simulink model "Experiment_3_cs"  (Simulink 8.4)
settings: Solver=ode5  SolverMode=SingleTasking  StartTime=0.0  StopTime=inf  FixedStep=1/100  RelTol=1e-3
PreLoadFcn:
  | mbxruntime.callbacks.PreLoadFcn(bdroot);
PostLoadFcn:
  | mbxruntime.callbacks.PostLoadFcn(bdroot);
InitFcn:
  | mbxruntime.callbacks.InitFcn(bdroot);
StartFcn:
  | mbxruntime.callbacks.StartFcn(bdroot);
StopFcn:
  | mbxruntime.callbacks.StopFcn(bdroot);
undefined symbols (not defined in the file or in its folder): dfreq, gray, Rec, SDTV, strel
libraries: simulink x88, PreScanSimulinkLibrary x24, simulink_extras x22, visiontextngfix x15, visionconversions x3, PreScanUsefulBlocks x3, visionsinks x2, simulink_need_slupdate x2, visionstatistics x1, visionmorphops x1, visionanalysis x1
(part 2 of 12)

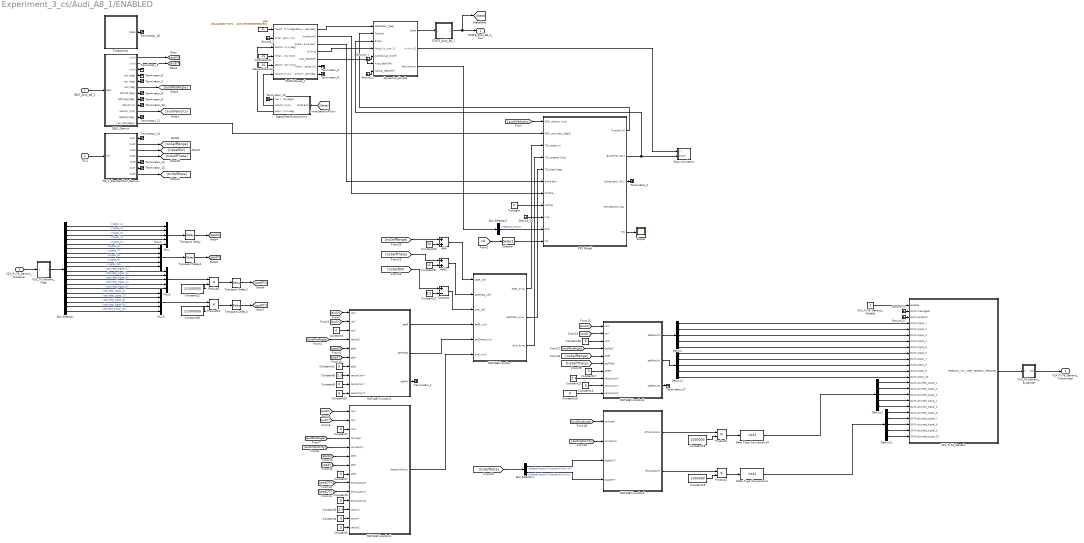
== system Experiment_3_cs/Audi_A8_1/ENABLED ==
  SELF_Audi_A8_1 : Inport  Tag=inport/SelfPort  OutDataTypeStr=Bus: PRESCAN_SELFSENSORDATA  PortDimensions=1  SampleTime=1/100  BusOutputAsStruct=on
  TIS_1 : Inport  Tag=inport/TIS  Port=2  OutDataTypeStr=Bus: PRESCAN_SCANNERSENSOR_MESSAGE  PortDimensions=5  SampleTime=1/50  BusOutputAsStruct=on
  V2X_Rx76_Generic_Receiver : Inport  Tag=inport/plugin/sfun_V2X_Generic_Receiver  Port=3  BusOutputAsStruct=on
  Add : Sum
  Add1 : Sum
  Bus Selector : BusSelector  OutputSignals=DATA.signal_1,DATA.signal_2,DATA.signal_3,DATA.signal_4,DATA.signal_5,DATA.signal_6,DATA.signal_7,DATA.signal_8,DATA.signal_9,DATA.signal_10,DATA.discrete_signal_1,DATA.discrete_signal_2,DATA.discrete_signal_3,DATA.discrete_signal_4,DATA.discrete_signal_5,DATA.discrete_signal_6,DATA.discrete_signal_7,DATA.discrete_signal_8,DATA.discrete_signal_9,DATA.discrete_signal_10
  Bus Selector1 : BusSelector  OutputSignals=DopplerVelocityTranslationX[ms-1],DopplerVelocityTranslationY[ms-1]
  Bus Selector2 : BusSelector  OutputSignals=NEngine_[rpm]
  Constant{,1..2,4..7,9..11,14..17} (14 alike) : Constant  Value=0
  Constant12 : Constant  Value=1/1000000
  Constant13 : Constant  Value=2.3
  Constant18 : Constant  Value=1000000
  Constant19 : Constant  Value=1000000
  Constant20 : Constant  Value=10
  Constant21 : Constant  Value=15
  Constant22 : Constant  Value=0.5
  Constant28 : Constant  Value=1/1000000
  Constant3 : Constant  Value=2.3
  Constant8 : Constant  Value=2.3
  Data Type Conversion1 : DataTypeConversion  OutDataTypeStr=int32
  Data Type Conversion10 : DataTypeConversion  OutDataTypeStr=int32
  Demux{,1..3} (4 alike) : Demux  Outputs=5
  DesiredVelocity : Constant  Tag=DesiredVelocity  Value=15
  Dynamics_Simple : Subsystem  Tag=Simple_Vehicle_Dynamics  mask(PreScan Block: Simple Dynamics){Migrate=on, TimeStep=1/100, ComputationMode=Continuous_Time}
      mask prompts: Migrate "Migrate. During migration this block will be replaced by a newer one."; TimeStep "Auto assigned: Time Step [s]"; ComputationMode "Computation mode:"
      mask help:
      | The Simple Dynamics Model is selected in the GUI to simulate vehicle dynamics behavior.
      |
      | The Simple Dynamics Model is completely open to the user. The parameters of this model can be set in the Simple Dynamics dialog in the GUI.
      |
      | For more information, please click Help.
      mask init:
      | p = SimpleDyn_pars;
      settings: DeleteFcn=PreScanBlockDeleteFcn;
      mask Help: eval('openHelp(220)')
      mask Display:
      | image(imread('SimpleDyn.png'))
      | port_label('input', 1, '{\delta}_S_t_ _e_e_r [deg]','texmode','on')
      | port_label('input', 2, 'Throttle [%]')
      | port_label('input', 3, 'Brake Pres [bar]')
      | port_label('input', 4, 'V_0 [ms-1]','texmode','on')
      | port_label('input', 5, 'Auto=[0]/Manual=[1]')
      | port_label('input', 6, 'Auto_GearShift')
      | port_label('input', 7, 'Manual_GearShift')
      | port_label('output', 1, 'State')
      | port_label('output', 2, 'Vx [ms-1]')
      | port_label('output', 3, 'Perf Params')
  Ground_{1..5,26} (6 alike) : Ground
  InitialVelocity : Constant  Tag=InitialVelocity  Value=15
  MATLAB Function : MATLAB Function  TreatAsAtomicUnit=on
  MATLAB Function1 : MATLAB Function  TreatAsAtomicUnit=on
  MATLAB Function2 : MATLAB Function  TreatAsAtomicUnit=on
  MATLAB Function3 : MATLAB Function  TreatAsAtomicUnit=on
  MATLAB Function4 : MATLAB Function  TreatAsAtomicUnit=on
  Mux{,1..3} (4 alike) : Mux  Inputs=5
  PPS Model : Subsystem  mask(PPS Model){MaxSpeed=70, MaxBrakePressure=150, BrakeDelay=100, LaneWidth=3.5, TISMaxRange=40, TISMaxTheta=60, TISfreq=25, TISdet=32, Camfreq=50, Mainfreq=100, DisplaySwitch=on, DisplayFreq=25, RadarSwitch=on, RadarFreq=25}
      mask prompts: MaxSpeed "Vehicle cut-off speed [km/h]"; MaxBrakePressure "Maximum value of braking pressure available [bar]"; BrakeDelay "Braking system delay [ms]"; LaneWidth "Lane width [m]"; TISMaxRange "TIS maximum range [m]"; TISMaxTheta "TIS maximum theta [deg]"; TISfreq "TIS frequency [Hz]"; TISdet "Max. number of Radar detected objects [-]"; Camfreq "Camera frequency [Hz]"; Mainfreq "Compilation sheet frequency [Hz]"; DisplaySwitch "Show EGO parameters visualization"; DisplayFreq "EGO parameters visualization frequency [Hz]"; RadarSwitch "Show radar visualization"; RadarFreq "Radar frequency [Hz]"
      mask help: PreScan Experiment and Pedestrian Protection System parameters
      mask Help: eval('openHelp(8130)')
      mask Callback DisplaySwitch:
      | en = get_param(gcb,'MaskEnables');
      | switch get_param(gcb, 'DisplaySwitch')
      |     case 'off'
      |         en{12} = 'off';
      |     case 'on'
      |         en{12} = 'on';
      | end
      | set_param(gcb,'MaskEnables',en);
      mask Callback RadarSwitch:
      | en = get_param(gcb,'MaskEnables');
      | switch get_param(gcb, 'RadarSwitch')
      |     case 'off'
      |         en{14} = 'off';
      |     case 'on'
      |         en{14} = 'on';
      | end
      | set_param(gcb,'MaskEnables',en);
  PathFollower_1 : Subsystem  Tag=pathFollower  mask(PreScan Block: Path Follower){Migrate=on, FileName='Trajectory_2.mat', TunableSteeringGain=1, XShifting_wrt_COG=0}
      mask prompts: Migrate "Migrate. During migration this block will be replaced by a newer one."; FileName "Trajectory Name"; TunableSteeringGain "TunableSteeringGain [-]"; XShifting_wrt_COG "XShifting_wrt_COG [m]"
      mask help:
      | The Path Follower Model is selected in the GUI to simulate driver behavior.
      |
      | For more information, please click Help.
      mask init:
      | load(['trajectories/',eval(FileName)])
      | traject=trajectory';
      | 
      | Traj_x=traject(:,2);
      | Traj_y=traject(:,3);
      | Traj_z=traject(:,4);
      | Traj_vx=traject(:,8);
      | Traj_vy=traject(:,9);
      | Traj_vz=traject(:,10);
      mask Help: eval('openHelp(232)')
  Product{1..3,12} (4 alike) : Product
  SELF_Demux : Subsystem  Tag=demux/SelfPort  mask(PreScan Demux Block:){}
      mask help:
      | The SELF port shows (state) information of the actor itself. The outputs are position in the experiment's axis system and the GPS coordinates, and the object's absolute velocity and compass heading.
      |
      | For more information, please click Help.
      settings: DeleteFcn=PreScanBlockDeleteFcn;
      mask Help: eval('openHelp(462)')
      mask Display:
      | port_label('output',1,'x [m]')
      | port_label('output',2,'y [m]')
      | port_label('output',3,'z [m]','texmode','on')
      | port_label('output',4,'Rotx [deg]','texmode','on')
      | port_label('output',5,'Roty [deg]','texmode','on')
      | port_label('output',6,'Rotz [deg]','texmode','on')
      | port_label('output',7,'GPS lat [deg]','texmode','on')
      | port_label('output',8,'GPS long [deg]','texmode','on')
      | port_label('output',9,'GPS alt [m]','texmode','on')
      | port_label('output',10,'Velocity [m/s]')
      | port_label('output',11,'Heading [deg]')
      | port_label('output',12,'Yaw rate [deg/s]')
  STATE_Audi_A8_1 : Subsystem  Tag=mux/StatePort  Priority=0  LoadFcn=load PrescanStateActuatorData  mask(PreScan Sink Block: State){x0=58.689357757568359, y0=151.23704528808594, z0=0.55, Roll0=0, Pitch0=0, Yaw0=359.99999999999295, TimeStep=1/100}
      mask prompts: x0 "Ini x-position VEHICLE wrt GLOBAL axis system [m]"; y0 "Ini y-position VEHICLE wrt GLOBAL axis system [m]"; z0 "Ini z-position VEHICLE wrt GLOBAL axis system [m]"; Roll0 "Ini roll-angle BODY wrt VEHICLE axis system [deg]"; Pitch0 "Ini pitch-angle BODY wrt VEHICLE axis system [deg]"; Yaw0 "Ini yaw-angle VEHICLE wrt GLOBAL axis system [deg]"; TimeStep "Auto-Assigned: Upload Period [s]"
      mask help:
      | The Actor State contains a vector signal of size (9x1), containing the following signals:
      |
      | -  Position                  (x,y,z)                                     [m]
      | -  Velocity                  (vx,vy,vz)                               [m/s]
      | -  Angles                    (Roll, Pitch, Yaw)                   [rad]
      |
      | The Actor state is defined in the global axis system.
      | The state is superponed on the Initial position defined in the GUI.
      |
      | For more information, please click Help.
      settings: DeleteFcn=PreScanBlockDeleteFcn;
      mask Help: eval('openHelp(222)')
      mask Display: image(imread('State.png'))
  Scope : Scope
  Selector : Selector  InputPortWidth=5
  State2PathFollowerCnv : Subsystem  Tag=State2PFConnection/cnv
  Stop simulation : Subsystem
  Subtract : Sum  Inputs=+-
  TIS_1_StandardCoh_Demux : Subsystem  Tag=demux/TIS/StandardCoh  TreatAsAtomicUnit=on  mask(PreScan Demux Block: TIS){MAXMESSAGES=5}
      mask prompts: MAXMESSAGES "Number of Objects"
      mask Help: eval('openHelp(449)')
      mask Display:
      | port_label('input',1,'TIS')
      | port_label('output',1,'Beam ID [-]')
      | port_label('output',2,'Range [m]')
      | port_label('output',3,'DopplerVelocity [m/s]')
      | port_label('output',4,'{\theta} [deg]','texmode','on')
      | port_label('output',5,'{\phi} [deg]','texmode','on')
      | port_label('output',6,'Target ID [-]','texmode','on')
      | port_label('output',7,'TIS Data','texmode','on')
  Terminator_{1..16,27} (17 alike) : Terminator
  Trajectories : Subsystem  Tag=Trajectories  mask(PreScan Source Block: Trajectories){}
      mask help:
      | The Trajectory block contains the trajectories defined in the PreScan Experiment Editor. The output of the trajectory block is the (vehicle) State.
      |
      | For more information, please click Help.
      settings: DeleteFcn=PreScanBlockDeleteFcn;
      mask Help: eval('openHelp(312)')
      mask Display: image(imread('Trajectory.png'));
  Transport Delay{,1..3} (4 alike) : TransportDelay  DelayTime=0.75
  V2X_76_Generic_Expander : Subsystem  LoadFcn=addpath .\V2XPlugin; V2Xbusses;
  V2X_76_Generic_Filter : Subsystem
      mask Display: disp('[1]');
  V2X_Tx76_Generic : Subsystem
  V2X_Tx76_Generic_Enable : Constant  OutDataTypeStr=Inherit: Inherit via back propagation
  pos : Constant  Tag=pos  Value=[58.689357757568359 151.23704528808594 359.99999999999295]
  STATE_Audi_A8_1_bus : Outport  Tag=outport/StatePort  OutDataTypeStr=Bus: PRESCAN_STATEACTUATORDATA  PortDimensions=1  SampleTime=1/100
  V2X_Tx76_Generic_Transmitter : Outport  Tag=outport/plugin/sfun_V2X_Generic_Transmitter  Port=2
  wires:
  SELF_Demux/12(yaw rate [deg/s]) -> PPS Model/2(EGO_yaw_rate_[deg/s])
  V2X_76_Generic_Filter/1(Filter_Out) -> Bus Selector/1
  Demux/1 -> V2X_Tx76_Generic/4(DATA.signal_1)
  Demux/2 -> V2X_Tx76_Generic/5(DATA.signal_2)
  Demux/3 -> V2X_Tx76_Generic/6(DATA.signal_3)
  Demux/4 -> V2X_Tx76_Generic/7(DATA.signal_4)
  Demux/5 -> V2X_Tx76_Generic/8(DATA.signal_5)
  Demux1/1 -> V2X_Tx76_Generic/9(DATA.signal_6)
  Demux1/2 -> V2X_Tx76_Generic/10(DATA.signal_7)
  Demux1/3 -> V2X_Tx76_Generic/11(DATA.signal_8)
  Demux1/4 -> V2X_Tx76_Generic/12(DATA.signal_9)
  Demux1/5 -> V2X_Tx76_Generic/13(DATA.signal_10)
  [audiX] -> MATLAB Function2/1(carX)
  [audiY] -> MATLAB Function2/2(carY)
  Constant1/1 -> MATLAB Function2/3(carZ)
  [audiRotAngle] -> MATLAB Function2/4(carRotZ)
  [audiX] -> MATLAB Function1/1(carX)
  [audiY] -> MATLAB Function1/2(carY)
  Constant2/1 -> MATLAB Function1/3(carZ)
  [audiRotAngle] -> MATLAB Function1/4(carAngle)
  [audiVelocity] -> MATLAB Function1/5(carVelocity)
  Constant3/1 -> MATLAB Function1/12(sensorX)
  Constant4/1 -> MATLAB Function1/13(sensorY)
  Constant5/1 -> MATLAB Function1/14(sensorZ)
  Constant6/1 -> MATLAB Function1/11(dTranslationZ)
  Constant7/1 -> MATLAB Function1/8(pedZ)
  Constant8/1 -> MATLAB Function2/8(sensorCorrX)
  Constant9/1 -> MATLAB Function2/9(sensorCorrY)
  Constant10/1 -> MATLAB Function2/10(sensorCorrZ)
  Constant11/1 -> MATLAB Function2/7(pedZ)
  [pedX] -> MATLAB Function2/5(pedX)
  [pedY] -> MATLAB Function2/6(pedY)
  [pedX] -> MATLAB Function1/6(pedX)
  [pedY] -> MATLAB Function1/7(pedY)
  [pedDTX] -> MATLAB Function1/9(dTranslationX)
  [pedDTY] -> MATLAB Function1/10(dTranslationY)
  Bus Selector2/1 -> PPS Model/10(RPM)  "<NEngine_[rpm]>"
  Selector/1 -> PPS Model/11(CD)
  [cd] -> Selector/1
  Constant/1 -> PPS Model/8(ind flag)
  PPS Model/5(TTC) -> Scope/1
  PPS Model/2(BrakePres [bar]) -> Dynamics_Simple/3(Brake), Stop simulation/2(brake)
  [audiVelocity] -> PPS Model/1(EGO_velocity [m/s])
  Constant12/1 -> Product1/2
  MATLAB Function/1(pedR_Array) -> PPS Model/3(TIS_range [m])
  MATLAB Function/2(pedTheta_Array) -> PPS Model/5(TIS_theta [deg])
  MATLAB Function/3(dVel_Array) -> PPS Model/4(TIS_rangedot [m/s])
  SELF_Demux/1(x [m]) -> [audiX]
  SELF_Demux/2(y [m]) -> [audiY]
  SELF_Demux/6(rotz [deg]) -> [audiRotAngle]
  SELF_Demux/10(velocity [m/s]) -> [audiVelocity]
  PathFollower_1/2(throttle [%]) -> PPS Model/7(throttle)
  PathFollower_1/3(brake pressure [bar]) -> PPS Model/6(brake dem)
  PPS Model/1(Throttle [%]) -> Dynamics_Simple/2(Throttle)
  Ground_26/1 -> PPS Model/9(img)
  Dynamics_Simple/2(Vx [m s-1]) -> Stop simulation/1(V)
  Dynamics_Simple/3(Perf_Params) -> Bus Selector2/1
  Constant13/1 -> MATLAB Function3/8(sensorCorrX)
  Constant14/1 -> MATLAB Function3/9(sensorCorrY)
  Constant15/1 -> MATLAB Function3/10(sensorCorrZ)
  Constant16/1 -> MATLAB Function3/3(carZ)
  Constant17/1 -> MATLAB Function3/7(pedPhi)
  Bus Selector1/1 -> MATLAB Function4/3(dopplerTX)  "<DopplerVelocityTranslationX[ms-1]>"
  Bus Selector1/2 -> MATLAB Function4/4(dopplerTY)  "<DopplerVelocityTranslationY[ms-1]>"
  [audiX] -> MATLAB Function3/1(carX)
  [audiY] -> MATLAB Function3/2(carY)
  [audiVelocity] -> MATLAB Function4/2(carVelocity)
  [audiRotAngle] -> MATLAB Function4/1(carAngle)
  [audiRotAngle] -> MATLAB Function3/4(carRotZ)
  MATLAB Function3/3(pedResultZ) -> Terminator_27/1
  MATLAB Function3/1(pedResultX) -> Demux/1
  MATLAB Function3/2(pedResultY) -> Demux1/1
  TIS_1_StandardCoh_Demux/2(Out2) -> [tisSelfRange]
  TIS_1_StandardCoh_Demux/3(Out3) -> [tisSelfDV]
  TIS_1_StandardCoh_Demux/4(Out4) -> [tisSelfTheta]
  TIS_1_StandardCoh_Demux/7(Out6) -> [tisSelfData]
  [tisSelfData] -> Bus Selector1/1
  [tisSelfRange] -> MATLAB Function3/5(pedR)
  [tisSelfTheta] -> MATLAB Function3/6(pedTheta)
  Bus Selector/1 -> Mux/1  "<signal_1>"
  Bus Selector/2 -> Mux/2  "<signal_2>"
  Bus Selector/3 -> Mux/3  "<signal_3>"
  Bus Selector/4 -> Mux/4  "<signal_4>"
  Bus Selector/5 -> Mux/5  "<signal_5>"
  Mux/1 -> Transport Delay/1
  Bus Selector/6 -> Mux1/1  "<signal_6>"
  Bus Selector/7 -> Mux1/2  "<signal_7>"
  Bus Selector/8 -> Mux1/3  "<signal_8>"
  Bus Selector/9 -> Mux1/4  "<signal_9>"
  Bus Selector/10 -> Mux1/5  "<signal_10>"
  Mux1/1 -> Transport Delay1/1
  Bus Selector/11 -> Mux2/1  "<discrete_signal_1>"
  Bus Selector/12 -> Mux2/2  "<discrete_signal_2>"
  Bus Selector/13 -> Mux2/3  "<discrete_signal_3>"
  Bus Selector/14 -> Mux2/4  "<discrete_signal_4>"
  Bus Selector/15 -> Mux2/5  "<discrete_signal_5>"
  Bus Selector/16 -> Mux3/1  "<discrete_signal_6>"
  Bus Selector/17 -> Mux3/2  "<discrete_signal_7>"
  Bus Selector/18 -> Mux3/3  "<discrete_signal_8>"
  Bus Selector/19 -> Mux3/4  "<discrete_signal_9>"
  Bus Selector/20 -> Mux3/5  "<discrete_signal_10>"
  Mux2/1 -> Product1/1
  Product1/1 -> Transport Delay2/1
  Constant28/1 -> Product12/2
  Mux3/1 -> Product12/1
  Product12/1 -> Transport Delay3/1
  Product3/1 -> Data Type Conversion10/1
  Constant18/1 -> Product3/2
  MATLAB Function4/1(dTranslationX) -> Product3/1
  Data Type Conversion10/1 -> Demux2/1
  Demux2/1 -> V2X_Tx76_Generic/14(DATA.discrete_signal_1)
  Demux2/2 -> V2X_Tx76_Generic/15(DATA.discrete_signal_2)
  Demux2/3 -> V2X_Tx76_Generic/16(DATA.discrete_signal_3)
  Demux2/4 -> V2X_Tx76_Generic/17(DATA.discrete_signal_4)
  Demux2/5 -> V2X_Tx76_Generic/18(DATA.discrete_signal_5)
  Demux3/1 -> V2X_Tx76_Generic/19(DATA.discrete_signal_6)
  Demux3/2 -> V2X_Tx76_Generic/20(DATA.discrete_signal_7)
  Demux3/3 -> V2X_Tx76_Generic/21(DATA.discrete_signal_8)
  Demux3/4 -> V2X_Tx76_Generic/22(DATA.discrete_signal_9)
  Demux3/5 -> V2X_Tx76_Generic/23(DATA.discrete_signal_10)
  Constant19/1 -> Product2/2
  Product2/1 -> Data Type Conversion1/1
  Data Type Conversion1/1 -> Demux3/1
  MATLAB Function4/2(dTranslationY) -> Product2/1
  [tisSelfDV] -> Subtract/1
  [tisSelfRange] -> Add/1
  Constant20/1 -> Add/2
  Add/1 -> MATLAB Function/1(pedR_self)
  [tisSelfTheta] -> Add1/1
  Constant21/1 -> Add1/2
  Add1/1 -> MATLAB Function/2(pedTheta_self)
  Constant22/1 -> Subtract/2
  Subtract/1 -> MATLAB Function/3(dVel_self)
  STATE_Audi_A8_1/1(StateBus) -> STATE_Audi_A8_1_bus/1, [State]
  SELF_Audi_A8_1/1 -> SELF_Demux/1(SELF)
  TIS_1/1 -> TIS_1_StandardCoh_Demux/1(TIS)
  pos/1 -> PathFollower_1/1(TrajOffset_x,y,Y [m,m,deg])
  InitialVelocity/1 -> PathFollower_1/4(Initial Velocity [m/s])
  DesiredVelocity/1 -> PathFollower_1/5(Desired Velocity [m/s])
  [State] -> State2PathFollowerCnv/1(State BUS)
  State2PathFollowerCnv/2(velocity [m/s]) -> PathFollower_1/6(velocity [m/s])
  State2PathFollowerCnv/3(position x,y,Y [m,m,deg]) -> PathFollower_1/3(position x,y,Y [m,m,deg])
  PathFollower_1/1(delta_steerwheel [deg]) -> Dynamics_Simple/1(DeltaSteer_[deg])
  PathFollower_1/4(v0 [m/s]) -> Dynamics_Simple/4(Initial_Vx_[ms-1])
  PathFollower_1/5(Auto_GearShift) -> Dynamics_Simple/6(Auto_GearShift)
  Dynamics_Simple/1(State) -> STATE_Audi_A8_1/1(State)
  V2X_Tx76_Generic_Enable/1 -> V2X_Tx76_Generic/1(Enabled)
  V2X_Tx76_Generic/1(PRESCAN_V2X_USER_GENERIC_MESSAGE) -> V2X_76_Generic_Expander/1(In)
  V2X_76_Generic_Expander/1(Out) -> V2X_Tx76_Generic_Transmitter/1
  V2X_Rx76_Generic_Receiver/1 -> V2X_76_Generic_Filter/1(Filter_In)
  Ground_1/1 -> Dynamics_Simple/5(AutoManual_OnOff)
  Ground_2/1 -> Dynamics_Simple/7(Manual_GearShift)
  MATLAB Function2/3(pedPhi) -> Terminator_1/1
  PPS Model/3(BrakeLights (3x1)) -> Terminator_2/1
  Ground_3/1 -> PathFollower_1/2(ActorOffset_Left(+) / Right(-) [m])
  PathFollower_1/6(Actor/Traj_distance [m]) -> Terminator_3/1
  PathFollower_1/7(Actor/Traj_angle [deg]) -> Terminator_4/1
  SELF_Demux/3(z [m]) -> Terminator_5/1
  SELF_Demux/4(rotx [deg]) -> Terminator_6/1
  SELF_Demux/5(roty [deg]) -> Terminator_7/1
  SELF_Demux/7(GPS lat [deg]) -> Terminator_8/1
  SELF_Demux/8(GPS long [deg]) -> Terminator_9/1
  SELF_Demux/9(GPS alt [m]) -> Terminator_10/1
  SELF_Demux/11(heading [deg]) -> Terminator_11/1
  State2PathFollowerCnv/1(Yaw rate [deg/s]) -> Terminator_12/1
  TIS_1_StandardCoh_Demux/1(Out1) -> Terminator_13/1
  TIS_1_StandardCoh_Demux/5(Out5) -> Terminator_14/1
  TIS_1_StandardCoh_Demux/6(Out7) -> Terminator_15/1
  Trajectories/1(State) -> Terminator_16/1
  Ground_4/1 -> V2X_Tx76_Generic/2(DATA.messageID)
  Ground_5/1 -> V2X_Tx76_Generic/3(DATA.senderID)
  MATLAB Function2/1(pedR) -> MATLAB Function/4(pedR_rcvd)
  MATLAB Function2/2(pedTheta) -> MATLAB Function/5(pedTheta_rcvd)
  MATLAB Function1/1(dopplerVelocity) -> MATLAB Function/6(dVel_rcvd)
  Transport Delay/1 -> [pedX]
  Transport Delay1/1 -> [pedY]
  Transport Delay2/1 -> [pedDTX]
  Transport Delay3/1 -> [pedDTY]

== system Experiment_3_cs/BMW_Z3_1/DISABLED ==
  SELF_BMW_Z3_1 : Inport  Tag=inport/SelfPort  OutDataTypeStr=Bus: PRESCAN_SELFSENSORDATA  PortDimensions=1  SampleTime=1/100  BusOutputAsStruct=on
  TIS_2 : Inport  Tag=inport/TIS  Port=2  OutDataTypeStr=Bus: PRESCAN_SCANNERSENSOR_MESSAGE  PortDimensions=5  SampleTime=1/50  BusOutputAsStruct=on
  V2X_Rx77_Generic_Receiver : Inport  Tag=inport/plugin/sfun_V2X_Generic_Receiver  Port=3  BusOutputAsStruct=on
  GND1 : Subsystem
  GND2 : Ground
  TRM1 : Terminator
  TRM2 : Terminator
  TRM3 : Terminator
  STATE_BMW_Z3_1_bus : Outport  Tag=outport/StatePort  OutDataTypeStr=Bus: PRESCAN_STATEACTUATORDATA  PortDimensions=1  SampleTime=1/100
  V2X_Tx77_Generic_Transmitter : Outport  Tag=outport/plugin/sfun_V2X_Generic_Transmitter  Port=2
  wires:
  SELF_BMW_Z3_1/1 -> TRM1/1
  TIS_2/1 -> TRM2/1
  V2X_Rx77_Generic_Receiver/1 -> TRM3/1
  GND1/1(bus) -> STATE_BMW_Z3_1_bus/1
  GND2/1 -> V2X_Tx77_Generic_Transmitter/1

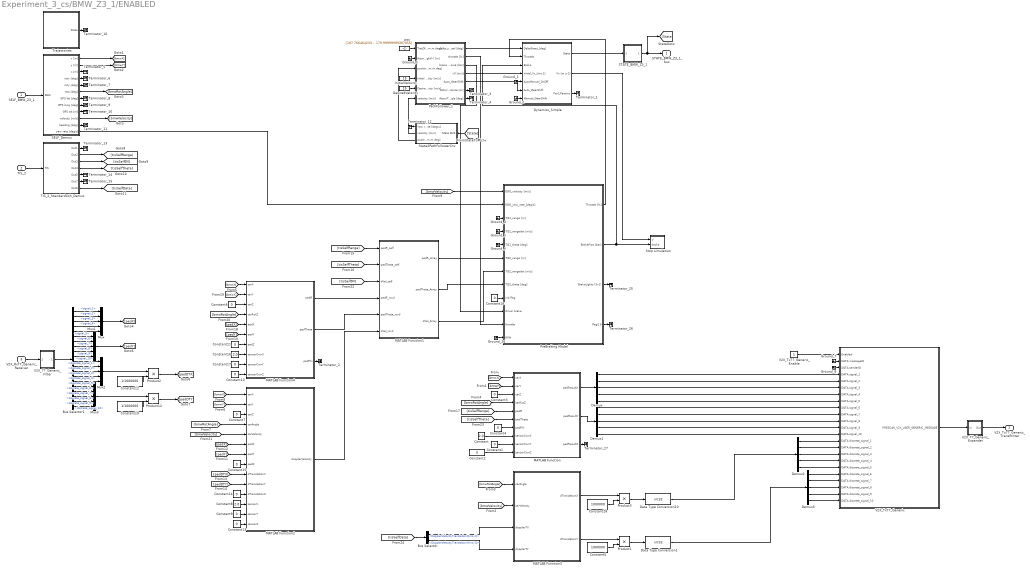
== system Experiment_3_cs/BMW_Z3_1/ENABLED ==
  SELF_BMW_Z3_1 : Inport  Tag=inport/SelfPort  OutDataTypeStr=Bus: PRESCAN_SELFSENSORDATA  PortDimensions=1  SampleTime=1/100  BusOutputAsStruct=on
  TIS_2 : Inport  Tag=inport/TIS  Port=2  OutDataTypeStr=Bus: PRESCAN_SCANNERSENSOR_MESSAGE  PortDimensions=5  SampleTime=1/50  BusOutputAsStruct=on
  V2X_Rx77_Generic_Receiver : Inport  Tag=inport/plugin/sfun_V2X_Generic_Receiver  Port=3  BusOutputAsStruct=on
  Bus Selector : BusSelector  OutputSignals=DopplerVelocityTranslationX[ms-1],DopplerVelocityTranslationY[ms-1]
  Bus Selector1 : BusSelector  OutputSignals=DATA.signal_1,DATA.signal_2,DATA.signal_3,DATA.signal_4,DATA.signal_5,DATA.signal_6,DATA.signal_7,DATA.signal_8,DATA.signal_9,DATA.signal_10,DATA.discrete_signal_1,DATA.discrete_signal_2,DATA.discrete_signal_3,DATA.discrete_signal_4,DATA.discrete_signal_5,DATA.discrete_signal_6,DATA.discrete_signal_7,DATA.discrete_signal_8,DATA.discrete_signal_9,DATA.discrete_signal_10
  Constant : Constant  Value=2.0
  Constant{1..4,6..7,9..11,13..15,17..18} (14 alike) : Constant  Value=0
  Constant12 : Constant  Value=1/1000000
  Constant16 : Constant  Value=2.0
  Constant19 : Constant  Value=1/1000000
  Constant28 : Constant  Value=1000000
  Constant5 : Constant  Value=1000000
  Constant8 : Constant  Value=2.0
  Data Type Conversion1 : DataTypeConversion  OutDataTypeStr=int32
  Data Type Conversion10 : DataTypeConversion  OutDataTypeStr=int32
  Demux{,1..3} (4 alike) : Demux  Outputs=5
  DesiredVelocity : Constant  Tag=DesiredVelocity  Value=15
  Dynamics_Simple : Subsystem  Tag=Simple_Vehicle_Dynamics  mask(PreScan Block: Simple Dynamics){Migrate=on, TimeStep=1/100, ComputationMode=Continuous_Time}
      mask prompts: Migrate "Migrate. During migration this block will be replaced by a newer one."; TimeStep "Auto assigned: Time Step [s]"; ComputationMode "Computation mode:"
      mask help:
      | The Simple Dynamics Model is selected in the GUI to simulate vehicle dynamics behavior.
      |
      | The Simple Dynamics Model is completely open to the user. The parameters of this model can be set in the Simple Dynamics dialog in the GUI.
      |
      | For more information, please click Help.
      mask init:
      | p = SimpleDyn_pars;
      settings: DeleteFcn=PreScanBlockDeleteFcn;
      mask Help: eval('openHelp(220)')
      mask Display:
      | image(imread('SimpleDyn.png'))
      | port_label('input', 1, '{\delta}_S_t_ _e_e_r [deg]','texmode','on')
      | port_label('input', 2, 'Throttle [%]')
      | port_label('input', 3, 'Brake Pres [bar]')
      | port_label('input', 4, 'V_0 [ms-1]','texmode','on')
      | port_label('input', 5, 'Auto=[0]/Manual=[1]')
      | port_label('input', 6, 'Auto_GearShift')
      | port_label('input', 7, 'Manual_GearShift')
      | port_label('output', 1, 'State')
      | port_label('output', 2, 'Vx [ms-1]')
      | port_label('output', 3, 'Perf Params')
  Ground_{1..8,26} (9 alike) : Ground
  InitialVelocity : Constant  Tag=InitialVelocity  Value=15
  MATLAB Function : MATLAB Function  TreatAsAtomicUnit=on
  MATLAB Function1 : MATLAB Function  TreatAsAtomicUnit=on
  MATLAB Function2 : MATLAB Function  TreatAsAtomicUnit=on
  MATLAB Function3 : MATLAB Function  TreatAsAtomicUnit=on
  MATLAB Function4 : MATLAB Function  TreatAsAtomicUnit=on
  Mux{,1..3} (4 alike) : Mux  Inputs=5
  PathFollower_1 : Subsystem  Tag=pathFollower  mask(PreScan Block: Path Follower){Migrate=on, FileName='Trajectory_1.mat', TunableSteeringGain=1, XShifting_wrt_COG=0}
      mask prompts: Migrate "Migrate. During migration this block will be replaced by a newer one."; FileName "Trajectory Name"; TunableSteeringGain "TunableSteeringGain [-]"; XShifting_wrt_COG "XShifting_wrt_COG [m]"
      mask help:
      | The Path Follower Model is selected in the GUI to simulate driver behavior.
      |
      | For more information, please click Help.
      mask init:
      | load(['trajectories/',eval(FileName)])
      | traject=trajectory';
      | 
      | Traj_x=traject(:,2);
      | Traj_y=traject(:,3);
      | Traj_z=traject(:,4);
      | Traj_vx=traject(:,8);
      | Traj_vy=traject(:,9);
      | Traj_vz=traject(:,10);
      mask Help: eval('openHelp(232)')
  PreBraking Model : Subsystem  mask(PreBraking Model){MaxBrakePressure=150, BrakingPercent=0.4, LaneWidth=3.5, TISMaxRange=[150 30], TISMaxTheta=[9 80], Tblock=1/100, Tsensor=[1/25 1/25], TISdet=[32 32], DisplaySwitch=on, DisplayFreq=25, RadarSwitch=on, RadarFreq=25}
      mask prompts: MaxBrakePressure "Maximum value of braking pressure [bar]"; BrakingPercent "Part of maximum braking pressure to use when partial braking [-]"; LaneWidth "Lane width [m]"; TISMaxRange "TIS maximum range (TIS1 and TIS2) [m]"; TISMaxTheta "TIS maximum theta angle (TIS1 and TIS2) [deg]"; Tblock "Target update rate of the compilation sheet [s]"; Tsensor "TIS update rate (TIS1 and TIS2) [s]"; TISdet "TIS max. objects to detect (TIS1 and TIS 2) [-]"; DisplaySwitch "Show EGO parameters visualization"; DisplayFreq "EGO parameters visualization frequency [Hz]"; RadarSwitch "Show radar visualization"; RadarFreq "Radar frequency [Hz]"
      mask help:
      | - intended to reduce speed of predicted collision,
      | - warns the driver and gives him more time to react,
      | - uses information from the state block
      |   and two independent TIS sensors,
      | - the system outputs are:
      |  = throttle and brake pressure (dynamics),
      |  = brake lights flags (light source visualisation animation)
      |  = the value of the warning flag.
      mask Help: eval('openHelp(1130)')
      mask Callback DisplaySwitch:
      | en = get_param(gcb,'MaskEnables');
      | switch get_param(gcb, 'DisplaySwitch')
      |     case 'off'
      |         en{10} = 'off';
      |     case 'on'
      |         en{10} = 'on';
      | end
      | set_param(gcb,'MaskEnables',en);
      mask Callback RadarSwitch:
      | en = get_param(gcb,'MaskEnables');
      | switch get_param(gcb, 'RadarSwitch')
      |     case 'off'
      |         en{12} = 'off';
      |     case 'on'
      |         en{12} = 'on';
      | end
      | set_param(gcb,'MaskEnables',en);
  Product{1..3,12} (4 alike) : Product
  SELF_Demux : Subsystem  Tag=demux/SelfPort  mask(PreScan Demux Block:){}
      mask help:
      | The SELF port shows (state) information of the actor itself. The outputs are position in the experiment's axis system and the GPS coordinates, and the object's absolute velocity and compass heading.
      |
      | For more information, please click Help.
      settings: DeleteFcn=PreScanBlockDeleteFcn;
      mask Help: eval('openHelp(462)')
      mask Display:
      | port_label('output',1,'x [m]')
      | port_label('output',2,'y [m]')
      | port_label('output',3,'z [m]','texmode','on')
      | port_label('output',4,'Rotx [deg]','texmode','on')
      | port_label('output',5,'Roty [deg]','texmode','on')
      | port_label('output',6,'Rotz [deg]','texmode','on')
      | port_label('output',7,'GPS lat [deg]','texmode','on')
      | port_label('output',8,'GPS long [deg]','texmode','on')
      | port_label('output',9,'GPS alt [m]','texmode','on')
      | port_label('output',10,'Velocity [m/s]')
      | port_label('output',11,'Heading [deg]')
      | port_label('output',12,'Yaw rate [deg/s]')
  STATE_BMW_Z3_1 : Subsystem  Tag=mux/StatePort  Priority=0  LoadFcn=load PrescanStateActuatorData  mask(PreScan Sink Block: State){x0=197.76646423339844, y0=155.00022888183594, z0=0.4784, Roll0=0, Pitch0=0, Yaw0=179.99999999387055, TimeStep=1/100}
      mask prompts: x0 "Ini x-position VEHICLE wrt GLOBAL axis system [m]"; y0 "Ini y-position VEHICLE wrt GLOBAL axis system [m]"; z0 "Ini z-position VEHICLE wrt GLOBAL axis system [m]"; Roll0 "Ini roll-angle BODY wrt VEHICLE axis system [deg]"; Pitch0 "Ini pitch-angle BODY wrt VEHICLE axis system [deg]"; Yaw0 "Ini yaw-angle VEHICLE wrt GLOBAL axis system [deg]"; TimeStep "Auto-Assigned: Upload Period [s]"
      mask help:
      | The Actor State contains a vector signal of size (9x1), containing the following signals:
      |
      | -  Position                  (x,y,z)                                     [m]
      | -  Velocity                  (vx,vy,vz)                               [m/s]
      | -  Angles                    (Roll, Pitch, Yaw)                   [rad]
      |
      | The Actor state is defined in the global axis system.
      | The state is superponed on the Initial position defined in the GUI.
      |
      | For more information, please click Help.
      settings: DeleteFcn=PreScanBlockDeleteFcn;
      mask Help: eval('openHelp(222)')
      mask Display: image(imread('State.png'))
  State2PathFollowerCnv : Subsystem  Tag=State2PFConnection/cnv
  Stop simulation : Subsystem
  TIS_2_StandardCoh_Demux : Subsystem  Tag=demux/TIS/StandardCoh  TreatAsAtomicUnit=on  mask(PreScan Demux Block: TIS){MAXMESSAGES=5}
      mask prompts: MAXMESSAGES "Number of Objects"
      mask Help: eval('openHelp(449)')
      mask Display:
      | port_label('input',1,'TIS')
      | port_label('output',1,'Beam ID [-]')
      | port_label('output',2,'Range [m]')
      | port_label('output',3,'DopplerVelocity [m/s]')
      | port_label('output',4,'{\theta} [deg]','texmode','on')
      | port_label('output',5,'{\phi} [deg]','texmode','on')
      | port_label('output',6,'Target ID [-]','texmode','on')
      | port_label('output',7,'TIS Data','texmode','on')
  Terminator_{1..16,25..27} (19 alike) : Terminator
  Trajectories : Subsystem  Tag=Trajectories  mask(PreScan Source Block: Trajectories){}
      mask help:
      | The Trajectory block contains the trajectories defined in the PreScan Experiment Editor. The output of the trajectory block is the (vehicle) State.
      |
      | For more information, please click Help.
      settings: DeleteFcn=PreScanBlockDeleteFcn;
      mask Help: eval('openHelp(312)')
      mask Display: image(imread('Trajectory.png'));
  V2X_77_Generic_Expander : Subsystem  LoadFcn=addpath .\V2XPlugin; V2Xbusses;
  V2X_77_Generic_Filter : Subsystem
      mask Display: disp('[1]');
  V2X_Tx77_Generic : Subsystem
  V2X_Tx77_Generic_Enable : Constant  OutDataTypeStr=Inherit: Inherit via back propagation
  pos : Constant  Tag=pos  Value=[197.76646423339844 155.00022888183594 179.99999999387055]
  STATE_BMW_Z3_1_bus : Outport  Tag=outport/StatePort  OutDataTypeStr=Bus: PRESCAN_STATEACTUATORDATA  PortDimensions=1  SampleTime=1/100
  V2X_Tx77_Generic_Transmitter : Outport  Tag=outport/plugin/sfun_V2X_Generic_Transmitter  Port=2
  wires:
  SELF_Demux/1(x [m]) -> [bmwX]
  SELF_Demux/2(y [m]) -> [bmwY]
  SELF_Demux/6(rotz [deg]) -> [bmwRotAngle]
  SELF_Demux/10(velocity [m/s]) -> [bmwVelocity]
  Constant/1 -> MATLAB Function/8(sensorCorrX)
  Constant1/1 -> MATLAB Function/9(sensorCorrY)
  Constant2/1 -> MATLAB Function/10(sensorCorrZ)
  Constant3/1 -> MATLAB Function/3(carZ)
  Constant4/1 -> MATLAB Function/7(pedPhi)
  Bus Selector/1 -> MATLAB Function3/3(dopplerTX)  "<DopplerVelocityTranslationX[ms-1]>"
  Bus Selector/2 -> MATLAB Function3/4(dopplerTY)  "<DopplerVelocityTranslationY[ms-1]>"
  [bmwX] -> MATLAB Function/1(carX)
  [bmwY] -> MATLAB Function/2(carY)
  [bmwVelocity] -> MATLAB Function3/2(carVelocity)
  [bmwRotAngle] -> MATLAB Function3/1(carAngle)
  [bmwRotAngle] -> MATLAB Function/4(carRotZ)
  MATLAB Function/3(pedResultZ) -> Terminator_27/1
  MATLAB Function/1(pedResultX) -> Demux/1
  [bmwX] -> MATLAB Function4/1(carX)
  [bmwY] -> MATLAB Function4/2(carY)
  Constant6/1 -> MATLAB Function4/3(carZ)
  [bmwRotAngle] -> MATLAB Function4/4(carRotZ)
  [bmwX] -> MATLAB Function2/1(carX)
  [bmwY] -> MATLAB Function2/2(carY)
  Constant7/1 -> MATLAB Function2/3(carZ)
  [bmwRotAngle] -> MATLAB Function2/4(carAngle)
  [bmwVelocity] -> MATLAB Function2/5(carVelocity)
  Constant8/1 -> MATLAB Function2/12(sensorX)
  Constant9/1 -> MATLAB Function2/13(sensorY)
  Constant13/1 -> MATLAB Function2/14(sensorZ)
  Constant14/1 -> MATLAB Function2/11(dTranslationZ)
  Constant15/1 -> MATLAB Function2/8(pedZ)
  Constant16/1 -> MATLAB Function4/8(sensorCorrX)
  Constant17/1 -> MATLAB Function4/9(sensorCorrY)
  Constant10/1 -> MATLAB Function4/10(sensorCorrZ)
  Constant11/1 -> MATLAB Function4/7(pedZ)
  [pedX] -> MATLAB Function4/5(pedX)
  [pedY] -> MATLAB Function4/6(pedY)
  [pedX] -> MATLAB Function2/6(pedX)
  [pedY] -> MATLAB Function2/7(pedY)
  [pedDTX] -> MATLAB Function2/9(dTranslationX)
  [pedDTY] -> MATLAB Function2/10(dTranslationY)
  Ground_26/1 -> PreBraking Model/12(RPM)
  PreBraking Model/1(Throttle [%]) -> Dynamics_Simple/2(Throttle)
  PreBraking Model/2(BrakePres [bar]) -> Dynamics_Simple/3(Brake), Stop simulation/2(brake)
  Demux/1 -> V2X_Tx77_Generic/4(DATA.signal_1)
  Demux/2 -> V2X_Tx77_Generic/5(DATA.signal_2)
  Demux/3 -> V2X_Tx77_Generic/6(DATA.signal_3)
  Demux/4 -> V2X_Tx77_Generic/7(DATA.signal_4)
  Demux/5 -> V2X_Tx77_Generic/8(DATA.signal_5)
  MATLAB Function/2(pedResultY) -> Demux1/1
  Demux1/1 -> V2X_Tx77_Generic/9(DATA.signal_6)
  Demux1/2 -> V2X_Tx77_Generic/10(DATA.signal_7)
  Demux1/3 -> V2X_Tx77_Generic/11(DATA.signal_8)
  Demux1/4 -> V2X_Tx77_Generic/12(DATA.signal_9)
  Demux1/5 -> V2X_Tx77_Generic/13(DATA.signal_10)
  TIS_2_StandardCoh_Demux/2(Out2) -> [tisSelfRange]
  TIS_2_StandardCoh_Demux/3(Out3) -> [tisSelfDV]
  TIS_2_StandardCoh_Demux/4(Out4) -> [tisSelfTheta]
  TIS_2_StandardCoh_Demux/7(Out6) -> [tisSelfData]
  [tisSelfRange] -> MATLAB Function1/1(pedR_self)
  [tisSelfTheta] -> MATLAB Function1/2(pedTheta_self)
  [tisSelfDV] -> MATLAB Function1/3(dVel_self)
  [tisSelfRange] -> MATLAB Function/5(pedR)
  [tisSelfTheta] -> MATLAB Function/6(pedTheta)
  [tisSelfData] -> Bus Selector/1
  Product3/1 -> Data Type Conversion10/1
  Constant28/1 -> Product3/2
  MATLAB Function3/1(dTranslationX) -> Product3/1
  Data Type Conversion10/1 -> Demux2/1
  Demux2/1 -> V2X_Tx77_Generic/14(DATA.discrete_signal_1)
  Demux2/2 -> V2X_Tx77_Generic/15(DATA.discrete_signal_2)
  Demux2/3 -> V2X_Tx77_Generic/16(DATA.discrete_signal_3)
  Demux2/4 -> V2X_Tx77_Generic/17(DATA.discrete_signal_4)
  Demux2/5 -> V2X_Tx77_Generic/18(DATA.discrete_signal_5)
  Demux3/1 -> V2X_Tx77_Generic/19(DATA.discrete_signal_6)
  Demux3/2 -> V2X_Tx77_Generic/20(DATA.discrete_signal_7)
  Demux3/3 -> V2X_Tx77_Generic/21(DATA.discrete_signal_8)
  Demux3/4 -> V2X_Tx77_Generic/22(DATA.discrete_signal_9)
  Demux3/5 -> V2X_Tx77_Generic/23(DATA.discrete_signal_10)
  Constant5/1 -> Product1/2
  Product1/1 -> Data Type Conversion1/1
  MATLAB Function3/2(dTranslationY) -> Product1/1
  Data Type Conversion1/1 -> Demux3/1
  V2X_77_Generic_Filter/1(Filter_Out) -> Bus Selector1/1
  Constant12/1 -> Product2/2
  Bus Selector1/1 -> Mux/1  "<signal_1>"
  Bus Selector1/2 -> Mux/2  "<signal_2>"
  Bus Selector1/3 -> Mux/3  "<signal_3>"
  Bus Selector1/4 -> Mux/4  "<signal_4>"
  Bus Selector1/5 -> Mux/5  "<signal_5>"
  Mux/1 -> [pedX]
  Bus Selector1/6 -> Mux1/1  "<signal_6>"
  Bus Selector1/7 -> Mux1/2  "<signal_7>"
  Bus Selector1/8 -> Mux1/3  "<signal_8>"
  Bus Selector1/9 -> Mux1/4  "<signal_9>"
  Bus Selector1/10 -> Mux1/5  "<signal_10>"
  Mux1/1 -> [pedY]
  Bus Selector1/11 -> Mux2/1  "<discrete_signal_1>"
  Bus Selector1/12 -> Mux2/2  "<discrete_signal_2>"
  Bus Selector1/13 -> Mux2/3  "<discrete_signal_3>"
  Bus Selector1/14 -> Mux2/4  "<discrete_signal_4>"
  Bus Selector1/15 -> Mux2/5  "<discrete_signal_5>"
  Bus Selector1/16 -> Mux3/1  "<discrete_signal_6>"
  Bus Selector1/17 -> Mux3/2  "<discrete_signal_7>"
  Bus Selector1/18 -> Mux3/3  "<discrete_signal_8>"
  Bus Selector1/19 -> Mux3/4  "<discrete_signal_9>"
  Bus Selector1/20 -> Mux3/5  "<discrete_signal_10>"
  Mux2/1 -> Product2/1
  Product2/1 -> [pedDTX]
  Constant19/1 -> Product12/2
  Mux3/1 -> Product12/1
  Product12/1 -> [pedDTY]
  Dynamics_Simple/2(Vx [m s-1]) -> Stop simulation/1(V)
  PathFollower_1/2(throttle [%]) -> PreBraking Model/11(throttle)
  PathFollower_1/3(brake pressure [bar]) -> PreBraking Model/10(driver brake)
  SELF_Demux/12(yaw rate [deg/s]) -> PreBraking Model/2(EGO_yaw_rate_[deg/s])
  Constant18/1 -> PreBraking Model/9(ind flag)
  PreBraking Model/3(BrakeLights (3x1)) -> Terminator_25/1
  PreBraking Model/4(flag2.6) -> Terminator_26/1
  [bmwVelocity] -> PreBraking Model/1(EGO_velocity [m/s])
  MATLAB Function1/1(pedR_Array) -> PreBraking Model/6(TIS2_range [m])
  MATLAB Function1/2(pedTheta_Array) -> PreBraking Model/8(TIS2_theta [deg])
  MATLAB Function1/3(dVel_Array) -> PreBraking Model/7(TIS2_rangedot [m/s])
  MATLAB Function4/1(pedR) -> MATLAB Function1/4(pedR_rcvd)
  MATLAB Function4/2(pedTheta) -> MATLAB Function1/5(pedTheta_rcvd)
  MATLAB Function2/1(dopplerVelocity) -> MATLAB Function1/6(dVel_rcvd)
  STATE_BMW_Z3_1/1(StateBus) -> STATE_BMW_Z3_1_bus/1, [State]
  SELF_BMW_Z3_1/1 -> SELF_Demux/1(SELF)
  TIS_2/1 -> TIS_2_StandardCoh_Demux/1(TIS)
  pos/1 -> PathFollower_1/1(TrajOffset_x,y,Y [m,m,deg])
  InitialVelocity/1 -> PathFollower_1/4(Initial Velocity [m/s])
  DesiredVelocity/1 -> PathFollower_1/5(Desired Velocity [m/s])
  [State] -> State2PathFollowerCnv/1(State BUS)
  State2PathFollowerCnv/2(velocity [m/s]) -> PathFollower_1/6(velocity [m/s])
  State2PathFollowerCnv/3(position x,y,Y [m,m,deg]) -> PathFollower_1/3(position x,y,Y [m,m,deg])
  PathFollower_1/1(delta_steerwheel [deg]) -> Dynamics_Simple/1(DeltaSteer_[deg])
  PathFollower_1/4(v0 [m/s]) -> Dynamics_Simple/4(Initial_Vx_[ms-1])
  PathFollower_1/5(Auto_GearShift) -> Dynamics_Simple/6(Auto_GearShift)
  Dynamics_Simple/1(State) -> STATE_BMW_Z3_1/1(State)
  V2X_Tx77_Generic_Enable/1 -> V2X_Tx77_Generic/1(Enabled)
  V2X_Tx77_Generic/1(PRESCAN_V2X_USER_GENERIC_MESSAGE) -> V2X_77_Generic_Expander/1(In)
  V2X_77_Generic_Expander/1(Out) -> V2X_Tx77_Generic_Transmitter/1
  V2X_Rx77_Generic_Receiver/1 -> V2X_77_Generic_Filter/1(Filter_In)
  Ground_1/1 -> Dynamics_Simple/5(AutoManual_OnOff)
  Ground_2/1 -> Dynamics_Simple/7(Manual_GearShift)
  Dynamics_Simple/3(Perf_Params) -> Terminator_1/1
  MATLAB Function4/3(pedPhi) -> Terminator_2/1
  Ground_3/1 -> PathFollower_1/2(ActorOffset_Left(+) / Right(-) [m])
  PathFollower_1/6(Actor/Traj_distance [m]) -> Terminator_3/1
  PathFollower_1/7(Actor/Traj_angle [deg]) -> Terminator_4/1
  Ground_4/1 -> PreBraking Model/3(TIS1_range [m])
  Ground_5/1 -> PreBraking Model/4(TIS1_rangedot [m/s])
  Ground_6/1 -> PreBraking Model/5(TIS1_theta [deg])
  SELF_Demux/3(z [m]) -> Terminator_5/1
  SELF_Demux/4(rotx [deg]) -> Terminator_6/1
  SELF_Demux/5(roty [deg]) -> Terminator_7/1
  SELF_Demux/7(GPS lat [deg]) -> Terminator_8/1
  SELF_Demux/8(GPS long [deg]) -> Terminator_9/1
  SELF_Demux/9(GPS alt [m]) -> Terminator_10/1
  SELF_Demux/11(heading [deg]) -> Terminator_11/1
  State2PathFollowerCnv/1(Yaw rate [deg/s]) -> Terminator_12/1
  TIS_2_StandardCoh_Demux/1(Out1) -> Terminator_13/1
  TIS_2_StandardCoh_Demux/5(Out5) -> Terminator_14/1
  TIS_2_StandardCoh_Demux/6(Out7) -> Terminator_15/1
  Trajectories/1(State) -> Terminator_16/1
  Ground_7/1 -> V2X_Tx77_Generic/2(DATA.messageID)
  Ground_8/1 -> V2X_Tx77_Generic/3(DATA.senderID)

== system Experiment_3_cs/CollisionDetection/DISABLED ==
  GND1 : Subsystem
  CollisionDetection : Outport  Tag=outport/CollisionDetection  OutDataTypeStr=Bus: PRESCAN_COLLISIONDETECTION_MESSAGE  PortDimensions=5  SampleTime=1/100
  wires:
  GND1/1(bus) -> CollisionDetection/1

== system Experiment_3_cs/CollisionDetection/ENABLED ==
  Sensor : S-Function  FunctionName=sfun_CollisionDetection  Parameters=detectableCollisions, timestep  EnableBusSupport=off  mask(PreScan Source Block: CollisionDetection){detectableCollisions=5, timestep=1/100}
      mask prompts: detectableCollisions "Max detectable collisions:"; timestep "MATLAB timestep:"
      mask help: Collision Detection can be used to detect collisions between PreScan components. For Collision Detection the actual component shape is taken into account, so it is not a bounding box approach.
      mask Help: eval('openHelp(811)')
      mask Display: image(imread('crash.jpg'))
  CollisionDetection : Outport  Tag=outport/CollisionDetection  OutDataTypeStr=Bus: PRESCAN_COLLISIONDETECTION_MESSAGE  PortDimensions=5  SampleTime=1/100
  wires:
  Sensor/1 -> CollisionDetection/1

== system Experiment_3_cs/Male_RegularAni_1/DISABLED ==
  SELF_Male_RegularAni_1 : Inport  Tag=inport/SelfPort  OutDataTypeStr=Bus: PRESCAN_SELFSENSORDATA  PortDimensions=1  SampleTime=1/100  BusOutputAsStruct=on
  GND1 : Subsystem
  GND2 : Subsystem
  TRM1 : Terminator
  STATE_Male_RegularAni_1_bus : Outport  Tag=outport/StatePort  OutDataTypeStr=Bus: PRESCAN_STATEACTUATORDATA  PortDimensions=1  SampleTime=1/100
  ANIM_Male_RegularAni_1 : Outport  Tag=outport/AnimationOutport  Port=2  OutDataTypeStr=Bus: PRESCAN_ANIMACTUATORDATA  PortDimensions=1  SampleTime=1/100
  wires:
  SELF_Male_RegularAni_1/1 -> TRM1/1
  GND1/1(bus) -> STATE_Male_RegularAni_1_bus/1
  GND2/1(bus) -> ANIM_Male_RegularAni_1/1

== system Experiment_3_cs/Male_RegularAni_1/ENABLED ==
  SELF_Male_RegularAni_1 : Inport  Tag=inport/SelfPort  OutDataTypeStr=Bus: PRESCAN_SELFSENSORDATA  PortDimensions=1  SampleTime=1/100  BusOutputAsStruct=on
  Animation : Subsystem  Tag=RunningHumanAnimation  mask(Prescan Conversion Block: Running Human Animation){MWS=1.95, WalkingScale=1.0, RunningScale=1.0, TimeStep=1/100}
      mask prompts: MWS "Maximum Walking Speed [m/s], above which the animation will switch to running mode."; WalkingScale "Walking mode scaling factor to sync the animation frames to the displacement."; RunningScale "Running mode scaling factor to sync the animation frames to the displacement."; TimeStep "Auto-Assigned: Upload Period [s]"
      mask help: The Running Human Animation block converts the State signal of a human into signals to properly control the animation.
      mask Help: eval('openHelp(239)');
      mask Display: image(imread('HumanAnimated.jpg'))
  SELF_Demux : Subsystem  Tag=demux/SelfPort  mask(PreScan Demux Block:){}
      mask help:
      | The SELF port shows (state) information of the actor itself. The outputs are position in the experiment's axis system and the GPS coordinates, and the object's absolute velocity and compass heading.
      |
      | For more information, please click Help.
      settings: DeleteFcn=PreScanBlockDeleteFcn;
      mask Help: eval('openHelp(462)')
      mask Display:
      | port_label('output',1,'x [m]')
      | port_label('output',2,'y [m]')
      | port_label('output',3,'z [m]','texmode','on')
      | port_label('output',4,'Rotx [deg]','texmode','on')
      | port_label('output',5,'Roty [deg]','texmode','on')
      | port_label('output',6,'Rotz [deg]','texmode','on')
      | port_label('output',7,'GPS lat [deg]','texmode','on')
      | port_label('output',8,'GPS long [deg]','texmode','on')
      | port_label('output',9,'GPS alt [m]','texmode','on')
      | port_label('output',10,'Velocity [m/s]')
      | port_label('output',11,'Heading [deg]')
      | port_label('output',12,'Yaw rate [deg/s]')
  STATE_Male_RegularAni_1 : Subsystem  Tag=mux/StatePort  Priority=0  LoadFcn=load PrescanStateActuatorData  mask(PreScan Sink Block: State){x0=126.19412994384766, y0=145.37350463867187, z0=0, Roll0=0, Pitch0=0, Yaw0=90.000000000651738, TimeStep=1/100}
      mask prompts: x0 "Ini x-position VEHICLE wrt GLOBAL axis system [m]"; y0 "Ini y-position VEHICLE wrt GLOBAL axis system [m]"; z0 "Ini z-position VEHICLE wrt GLOBAL axis system [m]"; Roll0 "Ini roll-angle BODY wrt VEHICLE axis system [deg]"; Pitch0 "Ini pitch-angle BODY wrt VEHICLE axis system [deg]"; Yaw0 "Ini yaw-angle VEHICLE wrt GLOBAL axis system [deg]"; TimeStep "Auto-Assigned: Upload Period [s]"
      mask help:
      | The Actor State contains a vector signal of size (9x1), containing the following signals:
      |
      | -  Position                  (x,y,z)                                     [m]
      | -  Velocity                  (vx,vy,vz)                               [m/s]
      | -  Angles                    (Roll, Pitch, Yaw)                   [rad]
      |
      | The Actor state is defined in the global axis system.
      | The state is superponed on the Initial position defined in the GUI.
      |
      | For more information, please click Help.
      settings: DeleteFcn=PreScanBlockDeleteFcn;
      mask Help: eval('openHelp(222)')
      mask Display: image(imread('State.png'))
  Terminator_{1..12} (12 alike) : Terminator
  Trajectories : Subsystem  Tag=Trajectories  mask(PreScan Source Block: Trajectories){}
      mask help:
      | The Trajectory block contains the trajectories defined in the PreScan Experiment Editor. The output of the trajectory block is the (vehicle) State.
      |
      | For more information, please click Help.
      settings: DeleteFcn=PreScanBlockDeleteFcn;
      mask Help: eval('openHelp(312)')
      mask Display: image(imread('Trajectory.png'));
  STATE_Male_RegularAni_1_bus : Outport  Tag=outport/StatePort  OutDataTypeStr=Bus: PRESCAN_STATEACTUATORDATA  PortDimensions=1  SampleTime=1/100
  ANIM_Male_RegularAni_1 : Outport  Tag=outport/AnimationOutport  Port=2  OutDataTypeStr=Bus: PRESCAN_ANIMACTUATORDATA  PortDimensions=1  SampleTime=1/100
  wires:
  STATE_Male_RegularAni_1/1(StateBus) -> STATE_Male_RegularAni_1_bus/1, Animation/1(In1)
  Animation/1(Out1) -> ANIM_Male_RegularAni_1/1
  SELF_Male_RegularAni_1/1 -> SELF_Demux/1(SELF)
  Trajectories/1(State) -> STATE_Male_RegularAni_1/1(State)
  SELF_Demux/1(x [m]) -> Terminator_1/1
  SELF_Demux/2(y [m]) -> Terminator_2/1
  SELF_Demux/3(z [m]) -> Terminator_3/1
  SELF_Demux/4(rotx [deg]) -> Terminator_4/1
  SELF_Demux/5(roty [deg]) -> Terminator_5/1
  SELF_Demux/6(rotz [deg]) -> Terminator_6/1
  SELF_Demux/7(GPS lat [deg]) -> Terminator_7/1
  SELF_Demux/8(GPS long [deg]) -> Terminator_8/1
  SELF_Demux/9(GPS alt [m]) -> Terminator_9/1
  SELF_Demux/10(velocity [m/s]) -> Terminator_10/1
  SELF_Demux/11(heading [deg]) -> Terminator_11/1
  SELF_Demux/12(yaw rate [deg/s]) -> Terminator_12/1

== system Experiment_3_cs/Nissan_Cabstar_1/DISABLED ==
  SELF_Nissan_Cabstar_1 : Inport  Tag=inport/SelfPort  OutDataTypeStr=Bus: PRESCAN_SELFSENSORDATA  PortDimensions=1  SampleTime=1/100  BusOutputAsStruct=on
  GND1 : Subsystem
  TRM1 : Terminator
  STATE_Nissan_Cabstar_1_bus : Outport  Tag=outport/StatePort  OutDataTypeStr=Bus: PRESCAN_STATEACTUATORDATA  PortDimensions=1  SampleTime=1/100
  wires:
  SELF_Nissan_Cabstar_1/1 -> TRM1/1
  GND1/1(bus) -> STATE_Nissan_Cabstar_1_bus/1

== system Experiment_3_cs/Nissan_Cabstar_1/ENABLED ==
  SELF_Nissan_Cabstar_1 : Inport  Tag=inport/SelfPort  OutDataTypeStr=Bus: PRESCAN_SELFSENSORDATA  PortDimensions=1  SampleTime=1/100  BusOutputAsStruct=on
  Dynamics_Empty : Subsystem  Tag=Dynamics_Empty
      mask Help: eval('openHelp(202)')
      mask Display: port_label('output', 1, 'State');text(0,0,' Empty\n')
  SELF_Demux : Subsystem  Tag=demux/SelfPort  mask(PreScan Demux Block:){}
      mask help:
      | The SELF port shows (state) information of the actor itself. The outputs are position in the experiment's axis system and the GPS coordinates, and the object's absolute velocity and compass heading.
      |
      | For more information, please click Help.
      settings: DeleteFcn=PreScanBlockDeleteFcn;
      mask Help: eval('openHelp(462)')
      mask Display:
      | port_label('output',1,'x [m]')
      | port_label('output',2,'y [m]')
      | port_label('output',3,'z [m]','texmode','on')
      | port_label('output',4,'Rotx [deg]','texmode','on')
      | port_label('output',5,'Roty [deg]','texmode','on')
      | port_label('output',6,'Rotz [deg]','texmode','on')
      | port_label('output',7,'GPS lat [deg]','texmode','on')
      | port_label('output',8,'GPS long [deg]','texmode','on')
      | port_label('output',9,'GPS alt [m]','texmode','on')
      | port_label('output',10,'Velocity [m/s]')
      | port_label('output',11,'Heading [deg]')
      | port_label('output',12,'Yaw rate [deg/s]')
  STATE_Nissan_Cabstar_1 : Subsystem  Tag=mux/StatePort  Priority=0  LoadFcn=load PrescanStateActuatorData  mask(PreScan Sink Block: State){x0=122.87779998779297, y0=144.38333129882813, z0=0.88, Roll0=0, Pitch0=0, Yaw0=0, TimeStep=1/100}
      mask prompts: x0 "Ini x-position VEHICLE wrt GLOBAL axis system [m]"; y0 "Ini y-position VEHICLE wrt GLOBAL axis system [m]"; z0 "Ini z-position VEHICLE wrt GLOBAL axis system [m]"; Roll0 "Ini roll-angle BODY wrt VEHICLE axis system [deg]"; Pitch0 "Ini pitch-angle BODY wrt VEHICLE axis system [deg]"; Yaw0 "Ini yaw-angle VEHICLE wrt GLOBAL axis system [deg]"; TimeStep "Auto-Assigned: Upload Period [s]"
      mask help:
      | The Actor State contains a vector signal of size (9x1), containing the following signals:
      |
      | -  Position                  (x,y,z)                                     [m]
      | -  Velocity                  (vx,vy,vz)                               [m/s]
      | -  Angles                    (Roll, Pitch, Yaw)                   [rad]
      |
      | The Actor state is defined in the global axis system.
      | The state is superponed on the Initial position defined in the GUI.
      |
      | For more information, please click Help.
      settings: DeleteFcn=PreScanBlockDeleteFcn;
      mask Help: eval('openHelp(222)')
      mask Display: image(imread('State.png'))
  Terminator_{1..12} (12 alike) : Terminator
  STATE_Nissan_Cabstar_1_bus : Outport  Tag=outport/StatePort  OutDataTypeStr=Bus: PRESCAN_STATEACTUATORDATA  PortDimensions=1  SampleTime=1/100
  wires:
  STATE_Nissan_Cabstar_1/1(StateBus) -> STATE_Nissan_Cabstar_1_bus/1
  SELF_Nissan_Cabstar_1/1 -> SELF_Demux/1(SELF)
  Dynamics_Empty/1(State) -> STATE_Nissan_Cabstar_1/1(State)
  SELF_Demux/1(x [m]) -> Terminator_1/1
  SELF_Demux/2(y [m]) -> Terminator_2/1
  SELF_Demux/3(z [m]) -> Terminator_3/1
  SELF_Demux/4(rotx [deg]) -> Terminator_4/1
  SELF_Demux/5(roty [deg]) -> Terminator_5/1
  SELF_Demux/6(rotz [deg]) -> Terminator_6/1
  SELF_Demux/7(GPS lat [deg]) -> Terminator_7/1
  SELF_Demux/8(GPS long [deg]) -> Terminator_8/1
  SELF_Demux/9(GPS alt [m]) -> Terminator_9/1
  SELF_Demux/10(velocity [m/s]) -> Terminator_10/1
  SELF_Demux/11(heading [deg]) -> Terminator_11/1
  SELF_Demux/12(yaw rate [deg/s]) -> Terminator_12/1

== system Experiment_3_cs/SELF_Actros_2541_1/DISABLED ==
  GND1 : Subsystem
  SELF_Actros_2541_1 : Outport  Tag=outport/SelfPort  OutDataTypeStr=Bus: PRESCAN_SELFSENSORDATA  PortDimensions=1  SampleTime=1/100
  wires:
  GND1/1(bus) -> SELF_Actros_2541_1/1
